simulink model "Sim_XY"  (R2016a)
settings: Solver=VariableStepAuto  StartTime=0.0  StopTime=10.0  RelTol=1e-3
values from neighbouring files (symbols this model uses):
  k_reg = 5.32    [Systemdesign_XY.m]    (also in Systemdesign_XY_Reduced.m = 10)
  k_s = double(subs(k_s,T_z,1))    [Systemdesign_XY.m]    (also in Systemdesign_XY_Reduced.m)
  T_n = T_sampl/2    (= 0.05)    [Systemdesign_XY.m]
  T_r = T_n*10    (= 0.5)    [Systemdesign_XY.m]    (also in Systemdesign_XY_Reduced.m = 0.2)
settings Model: Creator=Florian  LastModifiedBy=Florian

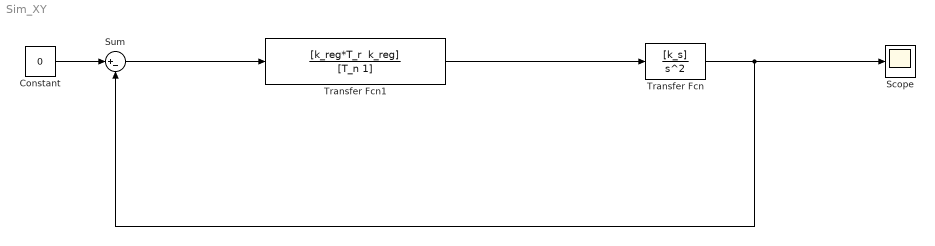
== system Sim_XY ==
  Constant : Constant  Value=0
  Scope : Scope
  Sum : Sum  Inputs=|+-
  Transfer Fcn : TransferFcn  Numerator=[k_s]  Denominator=[1 0 0]
  Transfer Fcn1 : TransferFcn  Numerator="[k_reg*T_r  k_reg]"  Denominator=[T_n 1]
  wires:
  Transfer Fcn/1 -> Scope/1, Sum/2
  Sum/1 -> Transfer Fcn1/1
  Constant/1 -> Sum/1
  Transfer Fcn1/1 -> Transfer Fcn/1
